simulink model "oscillating_leader_sim"  (R2024a)
settings: Solver=VariableStepAuto  StartTime=0.0  StopTime=10.0  RelTol=1e-3
model workspace (MAT data in the model file):
  modeVal = [0; 1; 2; 3]
settings Model: Creator=katiegildersleeve  LastModifiedBy=katiegildersleeve
settings DebuggingCC: UnderSpecifiedDimensionMsg=warning

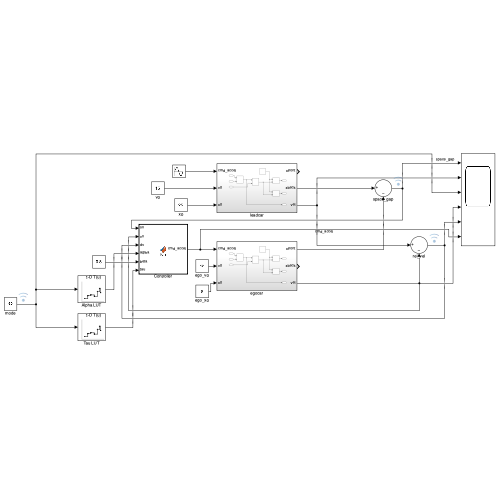
[thumbnail: Simulink's stored preview of the top-level diagram]
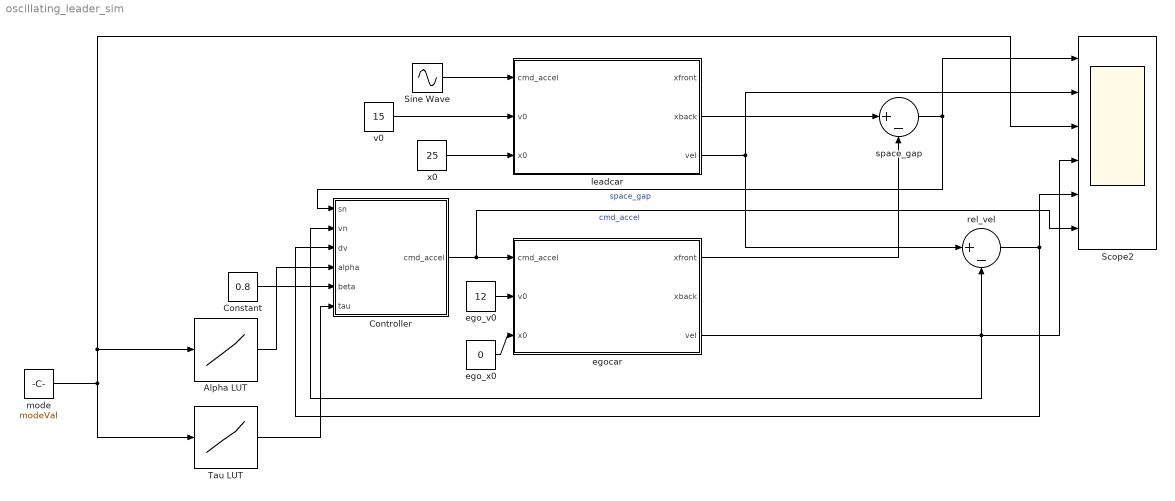
== system oscillating_leader_sim ==
  Alpha LUT : Lookup_n-D  NumberOfTableDimensions=1  BreakpointsForDimension1=[0 1 2 3]  Table=[0.75 0.75 1.0 0.25]  InterpMethod=Nearest  InternalRulePriority=Speed  RndMeth=Simplest
  Constant : Constant  Value=0.8
  Controller : MATLAB Function  TreatAsAtomicUnit=on
  Scope2 : Scope  NumInputPorts=6
  Sine Wave : Sin  SampleTime=0
  Tau LUT : Lookup_n-D  NumberOfTableDimensions=1  BreakpointsForDimension1=[0 1 2 3]  Table=[0.75 0.75 0.5 3.0]  InterpMethod=Nearest  InternalRulePriority=Speed  RndMeth=Simplest
  ego_v0 : Constant  Value=12
  ego_x0 : Constant  Value=0
  egocar : Subsystem
  leadcar : Subsystem
  mode : Constant  Value=modeVal
  rel_vel : Sum  Inputs=|+-
  space_gap : Sum  Inputs=|+-
  v0 : Constant  Value=15
  x0 : Constant  Value=25
  wires:
  v0/1 -> leadcar/2(v0)
  ego_v0/1 -> egocar/2(v0)
  egocar/3(vel) -> rel_vel/2, Controller/2(vn), Scope2/4
  leadcar/2(xback) -> space_gap/1
  space_gap/1 -> Scope2/1, Controller/1(sn)  "space_gap"
  egocar/1(xfront) -> space_gap/2
  Sine Wave/1 -> leadcar/1(cmd_accel)
  leadcar/3(vel) -> Scope2/2, rel_vel/1
  ego_x0/1 -> egocar/3(x0)
  rel_vel/1 -> Controller/3(dv), Scope2/5
  x0/1 -> leadcar/3(x0)
  Tau LUT/1 -> Controller/6(tau)
  Alpha LUT/1 -> Controller/4(alpha)
  mode/1 -> Tau LUT/1, Scope2/3, Alpha LUT/1
  Constant/1 -> Controller/5(beta)
  Controller/1(cmd_accel) -> Scope2/6, egocar/1(cmd_accel)  "cmd_accel"

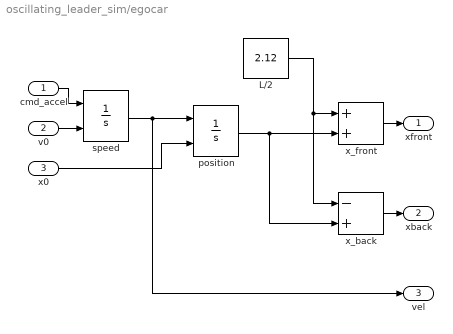
== system oscillating_leader_sim/egocar ==
  cmd_accel : Inport
  v0 : Inport  Port=2
  x0 : Inport  Port=3
  L/2 : Constant  Value=2.12
  position : Integrator  InitialConditionSource=external
  speed : Integrator  InitialConditionSource=external
  x_back : Sum  Inputs=-+
  x_front : Sum
  xfront : Outport
  xback : Outport  Port=2
  vel : Outport  Port=3
  wires:
  v0/1 -> speed/2
  x0/1 -> position/2
  cmd_accel/1 -> speed/1
  x_front/1 -> xfront/1
  x_back/1 -> xback/1
  position/1 -> x_back/2, x_front/2
  speed/1 -> vel/1, position/1
  L/2/1 -> x_back/1, x_front/1

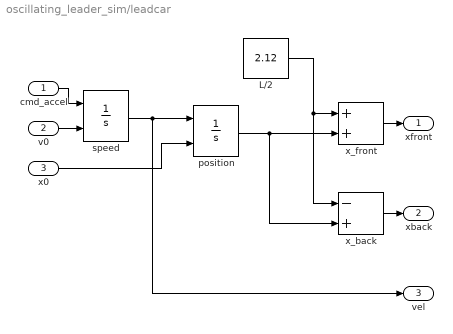
== system oscillating_leader_sim/leadcar ==
  cmd_accel : Inport
  v0 : Inport  Port=2
  x0 : Inport  Port=3
  L/2 : Constant  Value=2.12
  position : Integrator  InitialConditionSource=external
  speed : Integrator  InitialConditionSource=external
  x_back : Sum  Inputs=-+
  x_front : Sum
  xfront : Outport
  xback : Outport  Port=2
  vel : Outport  Port=3
  wires:
  v0/1 -> speed/2
  x0/1 -> position/2
  cmd_accel/1 -> speed/1
  x_front/1 -> xfront/1
  x_back/1 -> xback/1
  position/1 -> x_back/2, x_front/2
  speed/1 -> vel/1, position/1
  L/2/1 -> x_back/1, x_front/1

== matlab function oscillating_leader_sim/Controller ==
  data: sn input; vn input; dv input; cmd_accel output; alpha input; beta input; tau input
function cmd_accel = fcn(sn, vn, dv, alpha, beta, tau)
% sn   : geometric gap (lead back - ego front) [m]
% vn   : ego speed [m/s]
% dv   : v_lead - v_ego [m/s]   (NEG when ego is faster)

    % ---- force scalars in case any input arrives as a vector ----
    sn    = sn(1);
    vn    = vn(1);
    dv    = dv(1);
    alpha = alpha(1);
    beta  = beta   (1);
    tau   = tau   (1);

    % --- constants ---
    s_min = 5.0;     % standstill buffer [m]
    s_far = 50.0;    % use cruise control when gap > this [m]
    v_des = 25.0;    % desired cruise speed [m/s]
    a_min = -3.0;    % max braking  [m/s^2]
    a_max =  1.5;    % max accel    [m/s^2]

    % predeclare to fix output dimension
    a = 0.0;

    if sn > s_far
        % Far from leader: simple speed hold
        a = beta .* (v_des - vn);
    else
        % Within 50 m: time-gap + relative-velocity PD
        sn_eff = max(sn - s_min, 0.0);
        a = alpha .* (sn_eff - tau .* vn) + beta .* dv;

        % Emergency rule: inside buffer and still closing -> full brake
        if sn <= s_min && dv < 0
            a = a_min;
        end
    end

    % Clamp to actuator limits
    cmd_accel = min(max(a, a_min), a_max);
end
